simulink library "alloc_null"  (R2018b)
settings: Solver=VariableStepAuto  StartTime=0.0  StopTime=10.0  RelTol=1e-3
settings Model: Creator=Nick's PC  LastModifiedBy=Nick's PC

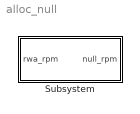
== system alloc_null ==
  Subsystem : Subsystem

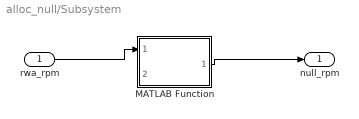
== system alloc_null/Subsystem ==
  rwa_rpm : Inport
  MATLAB Function : MATLAB Function  TreatAsAtomicUnit=on
  null_rpm : Outport
  wires:
  rwa_rpm/1 -> MATLAB Function/1(rwa_rpm)
  MATLAB Function/1(rwa_null_rpm) -> null_rpm/1

== matlab function alloc_null/Subsystem/MATLAB Function ==
  data: rwa_rpm input; rwa_null_rpm output; allocator input
function rwa_null_rpm = alloc_null(rwa_rpm,allocator)
%#codegen

h_targ = fswParams.allocator.h_targ_wheel_Nms;

nullvec = fswParams.allocator.nullvec;

h_rwa = rwa_rpm .* fswParams.constants.convert.RPM2RPS .* fswParams.allocator.inertia;

h_err = h_targ - h_rwa;

h_err_null_norm = h_err ./ nullvec;

rw_max = max(h_err_null_norm);

rw_min = min(h_err_null_norm);

null_multiplier = (rw_max + rw_min)/2;

rwa_optimal_null_Nm = -null_multiplier*nullvec;

rwa_null_rpm = (rwa_optimal_null_Nm ./ fswParams.allocator.inertia) .* fswParams.constants.convert.RPS2RPM;

end
